simulink model "ex_1"  (R2020b)
settings: Solver=ode23tb  StartTime=0.0  StopTime=20e3  MaxStep=1  RelTol=1e-3
libraries: component_lib x5, pid_lib x1
settings Model: Creator=maxjo65  LastModifiedBy=maxjo65

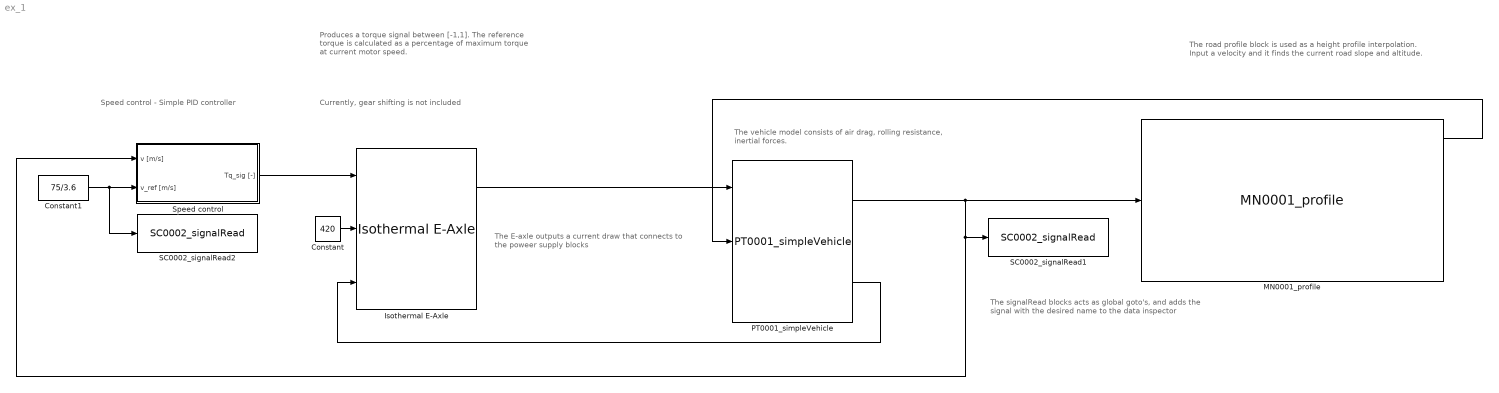
== system ex_1 ==
  note: The road profile block is used as a height profile interpolation.
      | Input a velocity and it finds the current road slope and altitude.
  note: The vehicle model consists of air drag, rolling resistance,
      | inertial forces.
  note: Currently, gear shifting is not included
  note: Produces a torque signal between [-1,1].
      |
      | The reference torque is calculated as a percentage of
      | maximum torque at current motor speed.
  note: Speed control - Simple PID controller
  note: The signalRead blocks acts as global goto's, and adds the signal with the desired name to the data inspector
  note: The E-axle outputs a current draw that connects
      | to the poweer supply blocks
  Constant : Constant  Value=420
  Constant1 : Constant  Value=75/3.6
  Isothermal E-Axle : component_lib/Isothermal E-Axle  n=2
  MN0001_profile : component_lib/Mission/MN0001_profile  profile=Munchen.mat  x0=0  N_lookahead=100
  PT0001_simpleVehicle : component_lib/Powertrain/PT0001_simpleVehicle  m=20e3  r_w=0.5  A_f=10  C_d=0.5  rho_air=1.225  c_r0=0.0060  c_r1=2.3e-7  gain=600  v0=75/3.6  x0=0
  SC0002_signalRead1 : component_lib/Data & Control/SC0002_signalRead  SigName=velocity
  SC0002_signalRead2 : component_lib/Data & Control/SC0002_signalRead  SigName=velocityReference
  Speed control : Subsystem
  wires:
  Constant/1 -> Isothermal E-Axle/2
  Isothermal E-Axle/1 -> PT0001_simpleVehicle/1
  PT0001_simpleVehicle/2 -> Isothermal E-Axle/3
  Speed control/1(Tq_sig [-]) -> Isothermal E-Axle/1
  Constant1/1 -> Speed control/2(v_ref [m/s]), SC0002_signalRead2/1
  MN0001_profile/1 -> PT0001_simpleVehicle/2
  PT0001_simpleVehicle/1 -> Speed control/1(v [m/s]), SC0002_signalRead1/1, MN0001_profile/1

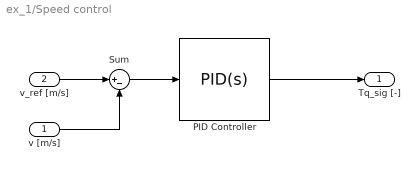
== system ex_1/Speed control ==
  v [m/s] : Inport
  v_ref [m/s] : Inport  Port=2
  PID Controller : pid_lib/PID Controller  Controller=PID  Form=Parallel  TimeDomain=Continuous-time  UseExternalTs=off  SampleTime=-1  IntegratorMethod=Forward Euler  FilterMethod=Forward Euler  ControllerParametersSource=internal  P=10  I=1e-1  D=0  UseFilter=on  N=100  TunerSelectOption=Transfer Function Based (PID Tuner App)  InitialConditionSource=internal  InitialConditionForIntegrator=0  InitialConditionForFilter=0  DifferentiatorICPrevScaledInput=0  ExternalReset=none  TrackingMode=off  Kt=1  LimitOutput=on  SatLimitsSource=internal  UpperSaturationLimit=1  LowerSaturationLimit=-1  LinearizeAsGain=on  AntiWindupMode=clamping  Kb=1  POutMin=[]  POutMax=[]  IOutMin=[]  IOutMax=[]  DOutMin=[]  DOutMax=[]  NOutMin=[]  NOutMax=[]  SumOutMin=[]  SumOutMax=[]  SaturationOutMin=[]  SaturationOutMax=[]  PParamMin=[]  PParamMax=[]  IParamMin=[]  IParamMax=[]  DParamMin=[]  DParamMax=[]  NParamMin=[]  NParamMax=[]  KbParamMin=[]  KbParamMax=[]  KtParamMin=[]  KtParamMax=[]  KbOutMin=[]  KbOutMax=[]  KtOutMin=[]  KtOutMax=[]  IntegratorOutMin=[]  IntegratorOutMax=[]  FilterOutMin=[]  FilterOutMax=[]  SumI1OutMin=[]  SumI1OutMax=[]  SumI2OutMin=[]  SumI2OutMax=[]  SumI3OutMin=[]  SumI3OutMax=[]  SumI4OutMin=[]  SumI4OutMax=[]  SumDOutMin=[]  SumDOutMax=[]  DifferentiatorOutMin=[]  DifferentiatorOutMax=[]  FilterDiffOutCoefMin=[]  FilterDiffOutCoefMax=[]  ReciprocalOutMin=[]  ReciprocalOutMax=[]  SumDenOutMin=[]  SumDenOutMax=[]  SumNumOutMin=[]  SumNumOutMax=[]  DivideOutMin=[]  DivideOutMax=[]  UdiffTsProdOutMin=[]  UdiffTsProdOutMax=[]  NTsProdOutMin=[]  NTsProdOutMax=[]  UintegralTsProdOutMin=[]  UintegralTsProdOutMax=[]  UngainTsProdOutMin=[]  UngainTsProdOutMax=[]  IntegratorContinuousStateAttributes=''  IntegratorStateMustResolveToSignalObject=off  IntegratorRTWStateStorageClass=Auto  FilterContinuousStateAttributes=''  FilterStateMustResolveToSignalObject=off  FilterRTWStateStorageClass=Auto  ParallelPVariant=InternalParameters  IdealPVariant=Disabled  IVariant=InternalParameters  DVariant=InternalParameters  IntegratorVariant=Continuous  SatVariant=Enabled  AWVariant=ContClampingParallel  PCopyVariant=Disabled  TRVariant=Disabled  FdbkBlocksVariant=Forward  IdealPFdbkVariant=Disabled  SatFdbkVariant=Disabled  DerivativeFilterVariant=ContFilter  NVariant=InternalParameters  NCopyVariant=Disabled  FilterICVariant=InternalICsFilter  IntegratorICVariant=InternalICs  ExternalResetVariant=Disabled  TRSumVariant=Passthrough  SumFdbkVariant=Disabled  SumVariant=Sum_PID  TsampFilterVariant=InternalTs  TsampNgainVariant=Passthrough  TsampIntegralVariant=Passthrough  ExternalSaturationOutDataTypeStr=Inherit: Same as second input
  Sum : Sum  Inputs=|+-
  Tq_sig [-] : Outport
  wires:
  PID Controller/1 -> Tq_sig [-]/1
  Sum/1 -> PID Controller/1
  v_ref [m/s]/1 -> Sum/1
  v [m/s]/1 -> Sum/2
